simulink model "parameter_tune"  (R2014b)
settings: Solver=FixedStepDiscrete  SolverMode=MultiTasking  StartTime=0.0  StopTime=inf  RelTol=1e-3
InitFcn:
  | TuneGain = 1
libraries: pixhawk_sllib x1
settings Model: SimulationMode=external  ExtModeBatchMode=on  TunableVars=TuneGain  TunableVarsStorageClass=Auto  Creator=skuznick  LastModifiedBy=darenlee
settings DataIOCC: SignalLoggingSaveFormat=ModelDataLogs
settings OptimizationCC: InlineParams=on  OptimizeModelRefInitCode=on  LifeSpan=1  MaxStackSize=64
settings DebuggingCC: MultiTaskDSMMsg=warning  MultiTaskCondExecSysMsg=none
settings HardwareCC: ProdLargestAtomicInteger=Long  ProdLargestAtomicFloat=Double  ProdEndianess=LittleEndian  ProdHWDeviceType=ARM Compatible->ARM Cortex
settings RTWCC: SystemTargetFile=ert.tlc  TemplateMakefile=ert_default_tmf  Description=Embedded Coder  GenerateReport=on  ProcessScript=ert_make_rtw_hook  Toolchain=Pixhawk Toolchain  IncludeHyperlinkInReport=on  LaunchReport=on  IncludeERTFirstTime=on  GenerateTraceInfo=on  GenerateTraceReport=on  GenerateTraceReportSl=on  GenerateTraceReportSf=on  GenerateTraceReportEml=on  GenerateCodeMetricsReport=on
settings CodeAppCC: IgnoreCustomStorageClasses=off
settings ERTTargetCC: ExtModeTransport=1  ExtModeStaticAllocSize=10000  ExtModeMexFile=ext_serial_win32_comm  ExtModeMexArgs=1 6 115200  ERTCustomFileTemplate=PX4_codertarget_file_process.tlc

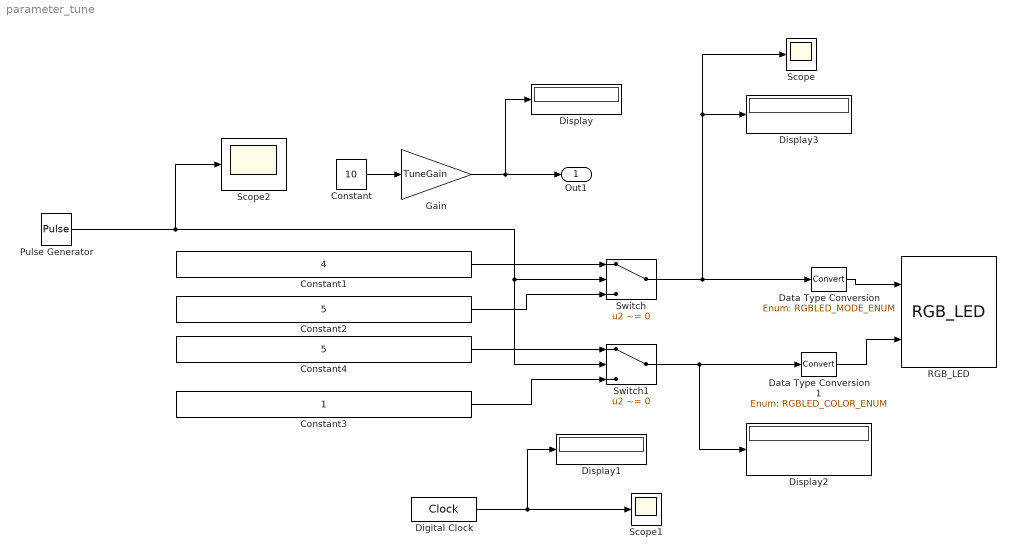
== system parameter_tune ==
  Constant : Constant  Value=10  SampleTime=0.1
  Constant1 : Constant  Value=4  OutDataTypeStr=int8
  Constant2 : Constant  Value=5  OutDataTypeStr=int8
  Constant3 : Constant  OutDataTypeStr=int8
  Constant4 : Constant  Value=5  OutDataTypeStr=int8
  Data Type Conversion : DataTypeConversion  OutDataTypeStr=Enum: RGBLED_MODE_ENUM
  Data Type Conversion1 : DataTypeConversion  OutDataTypeStr=Enum: RGBLED_COLOR_ENUM
  Digital Clock : DigitalClock  SampleTime=0.1
  Display{,1..3} (4 alike) : Display
  Gain : Gain  Gain=TuneGain
  Pulse Generator : DiscretePulseGenerator  PulseType=Time based  Period=6  PulseWidth=50
  RGB_LED : pixhawk_sllib/RGB_LED
  Scope : Scope
      settings: YMin=0  YMax=1
  Scope1 : Scope
      settings: YMin=9  YMax=18
  Scope2 : Scope
      settings: YMin=-0  YMax=2  SaveName=ScopeData2
  Switch : Switch  Criteria=u2 ~= 0  Threshold=1500
  Switch1 : Switch  Criteria=u2 ~= 0  Threshold=1500
  Out1 : Outport
  wires:
  Constant/1 -> Gain/1
  Gain/1 -> Display/1, Out1/1
  Switch/1 -> Scope/1, Display3/1, Data Type Conversion/1
  Switch1/1 -> Display2/1, Data Type Conversion1/1
  Constant1/1 -> Switch/1
  Constant2/1 -> Switch/3
  Constant4/1 -> Switch1/1
  Constant3/1 -> Switch1/3
  Pulse Generator/1 -> Scope2/1, Switch1/2, Switch/2
  Digital Clock/1 -> Display1/1, Scope1/1
  Data Type Conversion/1 -> RGB_LED/1
  Data Type Conversion1/1 -> RGB_LED/2
